simulink model "mavsim_chap2"  (R2018b)
settings: Solver=FixedStepDiscrete  StartTime=0.0  StopTime=1000  FixedStep=.1  RelTol=1e-3  EnableMultiTasking=on
InitFcn:
  | addpath('.')
undefined symbols (not defined in the file or in its folder): drawAircraft
libraries: simulink x6
settings Model: Creator=beard  LastModifiedBy=do
settings DataIOCC: LimitDataPoints=on  SaveFormat=Array  SignalLoggingSaveFormat=ModelDataLogs
settings OptimizationCC: ExpressionDepthLimit=2147483647  InitFltsAndDblsToZero=on  LifeSpan=inf
settings DebuggingCC: UnderspecifiedInitializationDetection=Classic  MergeDetectMultiDrivingBlocksExec=none  SolverPrmCheckMsg=warning  FcnCallInpInsideContextMsg=warning  AllowSymbolicDim=off  StateNameClashWarn=warning  SFUnexpectedBacktrackingDiag=warning  SFNoUnconditionalDefaultTransitionDiag=warning  SFExecutionAtInitializationDiag=none
settings HardwareCC: ProdBitPerPointer=32  ProdBitPerSizeT=32  ProdBitPerPtrDiffT=32  ProdLargestAtomicFloat=None  ProdIntDivRoundTo=Undefined  ProdEndianess=Unspecified  ProdWordSize=32  ProdHWDeviceType=32-bit Generic
settings ModelReferenceCC: PropagateSignalLabelsOutOfModel=off
settings SFSimCC: SimUseLocalCustomCode=off
settings RTWCC: RTWUseLocalCustomCode=off
settings CodeAppCC: StateflowObjectComments=on
settings GRTTargetCC: TargetLangStandard=C89/C90 (ANSI)  GeneratePreprocessorConditionals=Disable all  CombineOutputUpdateFcns=off  GRTInterface=on
settings ConfigComp: CovMetricSettings=dw  CovHtmlReporting=on  CovSaveCumulativeToWorkspaceVar=on  CovSaveSingleToWorkspaceVar=on  CovExternalEMLEnable=off  CovSFcnEnable=off

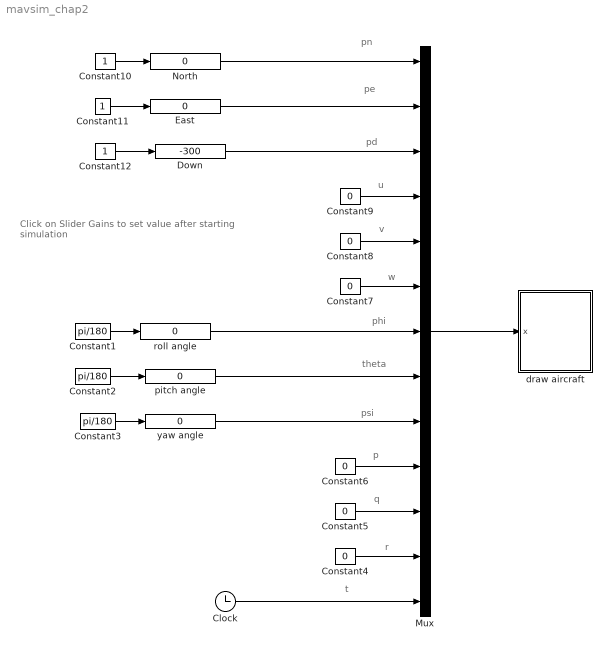
== system mavsim_chap2 ==
  note: t
  note: pn
  note: pe
  note: pd
  note: phi
  note: theta
  note: psi
  note: p
  note: q
  note: r
  note: u
  note: v
  note: w
  note: Click on Slider Gains to set value
      | after starting simulation
  Clock : Clock
  Constant1 : Constant  Value=pi/180
  Constant10 : Constant
  Constant11 : Constant
  Constant12 : Constant
  Constant2 : Constant  Value=pi/180
  Constant3 : Constant  Value=pi/180
  Constant{4..9} (6 alike) : Constant  Value=0
  Down : simulink/Math Operations/Slider Gain  gain=-300  low=-1000  high=0
  East : simulink/Math Operations/Slider Gain  gain=0  low=-1000  high=1000
  Mux : Mux  Inputs=13
  North : simulink/Math Operations/Slider Gain  gain=0  low=-900  high=900
  draw aircraft : Subsystem
      mask Display: image(imread('tv.jpg'))
  pitch angle : simulink/Math Operations/Slider Gain  gain=0  low=-180  high=180
  roll angle : simulink/Math Operations/Slider Gain  gain=0  low=-180  high=180
  "yaw angle " : simulink/Math Operations/Slider Gain  gain=0  low=-180  high=180
  wires:
  Mux/1 -> draw aircraft/1(x)
  roll angle/1 -> Mux/7
  Constant1/1 -> roll angle/1
  pitch angle/1 -> Mux/8
  Constant2/1 -> pitch angle/1
  "yaw angle "/1 -> Mux/9
  Constant3/1 -> "yaw angle "/1
  Constant4/1 -> Mux/12
  Constant5/1 -> Mux/11
  Constant6/1 -> Mux/10
  Constant7/1 -> Mux/6
  Constant8/1 -> Mux/5
  Constant9/1 -> Mux/4
  East/1 -> Mux/2
  Constant11/1 -> East/1
  Down/1 -> Mux/3
  Constant12/1 -> Down/1
  North/1 -> Mux/1
  Constant10/1 -> North/1
  Clock/1 -> Mux/13

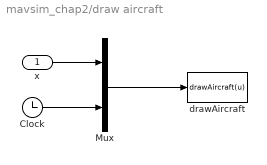
== system mavsim_chap2/draw aircraft ==
  x : Inport
  Clock : Clock
  Mux : Mux  Inputs=2
  drawAircraft : MATLABFcn  MATLABFcn=drawAircraft(u)  OutputDimensions=0  SampleTime=0.1
  wires:
  Mux/1 -> drawAircraft/1
  x/1 -> Mux/1
  Clock/1 -> Mux/2
